simulink model "ea_model"  (Simulink 8.8)
settings: Solver=ode23  StartTime=0.0  StopTime=10  MaxStep=.01  RelTol=1e-3  AbsTol=1e-3  EnableMultiTasking=on
undefined symbols (not defined in the file): i_smn0, L_s, M, p, psi_r_al_bet0, psi_Rmn0, psi_s_al_bet0, R_r, R_s, sigma, tau_r, tau_sigma
settings Model: Creator=Niels  LastModifiedBy=Niels  ExtModeTrigMode=oneshot  ExtModeArmWhenConnect=off
settings DataIOCC: LimitDataPoints=off  SaveOutput=off  SaveTime=off
settings OptimizationCC: BlockReduction=off  BooleanDataType=off  LifeSpan=auto
settings DebuggingCC: SaveWithParameterizedLinksMsg=none  SignalResolutionControl=TryResolveAllWithWarning  MultiTaskDSMMsg=warning  MultiTaskCondExecSysMsg=none  FcnCallInpInsideContextMsg=error  StateNameClashWarn=none  StrictBusMsg=None  SFUnexpectedBacktrackingDiag=error  SFNoUnconditionalDefaultTransitionDiag=error  SFExecutionAtInitializationDiag=warning
settings HardwareCC: ProdBitPerPointer=64  ProdBitPerSizeT=64  ProdBitPerPtrDiffT=64  ProdLargestAtomicFloat=Float  ProdIntDivRoundTo=Zero  ProdEndianess=LittleEndian  ProdWordSize=64  ProdHWDeviceType=Intel->x86-64 (Windows64)  TargetUnknown=on
settings GRTTargetCC: GeneratePreprocessorConditionals=Use local settings
settings ConfigComp: CovMetricSettings=dwe  CovHtmlReporting=off  CovSaveCumulativeToWorkspaceVar=off  CovSaveSingleToWorkspaceVar=off  CovExternalEMLEnable=on

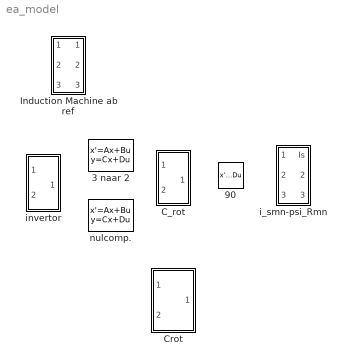
== system ea_model ==
  3 naar 2 : StateSpace  A=[]  B=[]  C=[]  D=K  X0=0  mask(Matrix gain){K=[2/3 -1/3 -1/3; 0 1/sqrt(3) -1/sqrt(3)]}
      mask prompts: K "Gain matrix:"
      mask help: Matrix Gain.
      mask Help: Multiplies input vector by entered matrix to produce output vector (y=Au).
      mask Display: disp('K')
  90 : StateSpace  A=[]  B=[]  C=[]  D=K  X0=0  mask(Matrix gain){K=[0 -1;1 0]}
      mask prompts: K "Gain matrix:"
      mask help: Matrix Gain.
      mask Help: Multiplies input vector by entered matrix to produce output vector (y=Au).
      mask Display: disp('K')
  C_rot : Subsystem
  Crot : Subsystem
  Induction Machine ab ref : Subsystem
  i_smn-psi_Rmn : Subsystem
  invertor : Subsystem
  nulcomp. : StateSpace  A=[]  B=[]  C=[]  D=K  X0=0  mask(Matrix gain){K=[1/3 1/3 1/3]}
      mask prompts: K "Gain matrix:"
      mask help: Matrix Gain.
      mask Help: Multiplies input vector by entered matrix to produce output vector (y=Au).
      mask Display: disp('K')

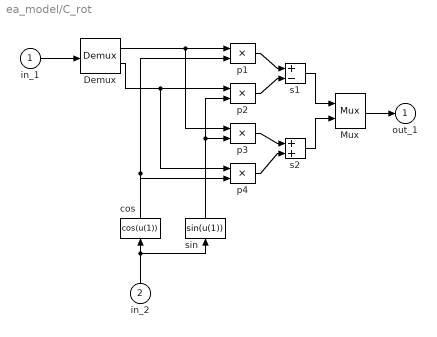
== system ea_model/C_rot ==
  in_1 : Inport
  in_2 : Inport  Port=2
  Demux : Demux  Outputs=2
  Mux : Mux  Inputs=2
  cos : Fcn  Expr=cos(u(1))
  p{1..4} (4 alike) : Product  SaturateOnIntegerOverflow=on  RndMeth=Zero  InputSameDT=on  OutDataTypeStr=Inherit: Same as first input
  s1 : Sum  Inputs=+-  SaturateOnIntegerOverflow=on  InputSameDT=on  OutDataTypeStr=Inherit: Same as first input
  s2 : Sum  SaturateOnIntegerOverflow=on  InputSameDT=on  OutDataTypeStr=Inherit: Same as first input
  sin : Fcn  Expr=sin(u(1))
  out_1 : Outport
  wires:
  s2/1 -> Mux/2
  s1/1 -> Mux/1
  p2/1 -> s1/2
  p3/1 -> s2/1
  p1/1 -> s1/1
  p4/1 -> s2/2
  in_2/1 -> cos/1, sin/1
  sin/1 -> p2/2, p3/2
  cos/1 -> p1/2, p4/2
  Demux/1 -> p1/1, p3/1
  Demux/2 -> p2/1, p4/1
  in_1/1 -> Demux/1
  Mux/1 -> out_1/1

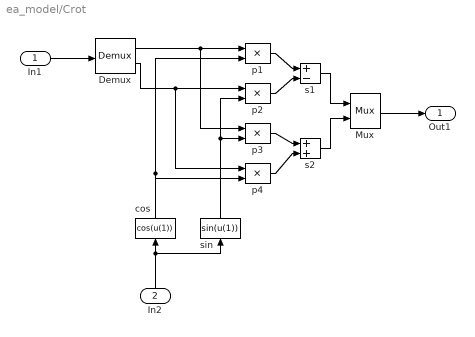
== system ea_model/Crot ==
  In1 : Inport
  In2 : Inport  Port=2
  Demux : Demux  Outputs=2
  Mux : Mux  Inputs=2
  cos : Fcn  Expr=cos(u(1))
  p{1..4} (4 alike) : Product  SaturateOnIntegerOverflow=on  RndMeth=Zero  InputSameDT=on  OutDataTypeStr=Inherit: Same as first input
  s1 : Sum  Inputs=+-  SaturateOnIntegerOverflow=on  InputSameDT=on  OutDataTypeStr=Inherit: Same as first input
  s2 : Sum  SaturateOnIntegerOverflow=on  InputSameDT=on  OutDataTypeStr=Inherit: Same as first input
  sin : Fcn  Expr=sin(u(1))
  Out1 : Outport
  wires:
  sin/1 -> p2/2, p3/2
  cos/1 -> p1/2, p4/2
  In2/1 -> cos/1, sin/1
  In1/1 -> Demux/1
  p2/1 -> s1/2
  s1/1 -> Mux/1
  Demux/1 -> p1/1, p3/1
  Mux/1 -> Out1/1
  Demux/2 -> p2/1, p4/1
  s2/1 -> Mux/2
  p3/1 -> s2/1
  p1/1 -> s1/1
  p4/1 -> s2/2

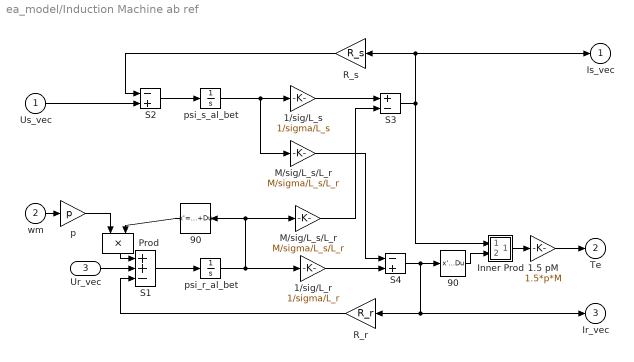
== system ea_model/Induction Machine ab ref ==
  Us_vec : Inport
  wm : Inport  Port=2
  Ur_vec : Inport  Port=3
  1.5 pM : Gain  Gain=1.5*p*M  SaturateOnIntegerOverflow=on  OutDataTypeStr=Inherit: Same as input  ParamDataTypeStr=Inherit: Same as input
  1/sig/L_r : Gain  Gain=1/sigma/L_r  SaturateOnIntegerOverflow=on  OutDataTypeStr=Inherit: Same as input  ParamDataTypeStr=Inherit: Same as input
  "1/sig/L_s " : Gain  Gain=1/sigma/L_s  SaturateOnIntegerOverflow=on  OutDataTypeStr=Inherit: Same as input  ParamDataTypeStr=Inherit: Same as input
  90 : StateSpace  A=[]  B=[]  C=[]  D=K  X0=0  mask(Matrix gain){K=[0 -1;1 0]}
      mask prompts: K "Gain matrix:"
      mask help: Matrix Gain.
      mask Help: Multiplies input vector by entered matrix to produce output vector (y=Au).
      mask Display: disp('K')
  "90 " : StateSpace  A=[]  B=[]  C=[]  D=K  X0=0  mask(Matrix gain){K=[0 -1;1 0]}
      mask prompts: K "Gain matrix:"
      mask help: Matrix Gain.
      mask Help: Multiplies input vector by entered matrix to produce output vector (y=Au).
      mask Display: disp('K')
  Inner Prod : Subsystem  mask(Dot Product){}
      mask help:
      | Inner (dot) product.
      | y=sum(u1.*u2)
      mask Help: Computes the inner (dot) product of the inputs: sum(u1.*u2).  The inputs are vectors of the same length. Output is a scalar.
      mask Display: disp('.\n')
  M/sig/L_s/L_r : Gain  Gain=M/sigma/L_s/L_r  SaturateOnIntegerOverflow=on  OutDataTypeStr=Inherit: Same as input  ParamDataTypeStr=Inherit: Same as input
  "M/sig/L_s/L_r " : Gain  Gain=M/sigma/L_s/L_r  SaturateOnIntegerOverflow=on  OutDataTypeStr=Inherit: Same as input  ParamDataTypeStr=Inherit: Same as input
  Prod : Product  SaturateOnIntegerOverflow=on  RndMeth=Zero  InputSameDT=on  OutDataTypeStr=Inherit: Same as first input
  R_r : Gain  Gain=R_r  SaturateOnIntegerOverflow=on  OutDataTypeStr=Inherit: Same as input  ParamDataTypeStr=Inherit: Same as input
  R_s : Gain  Gain=R_s  SaturateOnIntegerOverflow=on  OutDataTypeStr=Inherit: Same as input  ParamDataTypeStr=Inherit: Same as input
  S1 : Sum  Inputs=++-  SaturateOnIntegerOverflow=on  InputSameDT=on  OutDataTypeStr=Inherit: Same as first input
  S2 : Sum  Inputs=-+  SaturateOnIntegerOverflow=on  InputSameDT=on  OutDataTypeStr=Inherit: Same as first input
  S3 : Sum  Inputs=+-  SaturateOnIntegerOverflow=on  InputSameDT=on  OutDataTypeStr=Inherit: Same as first input
  S4 : Sum  Inputs=-+  SaturateOnIntegerOverflow=on  InputSameDT=on  OutDataTypeStr=Inherit: Same as first input
  p : Gain  Gain=p  SaturateOnIntegerOverflow=on  OutDataTypeStr=Inherit: Same as input  ParamDataTypeStr=Inherit: Same as input
  psi_r_al_bet : Integrator  InitialCondition=psi_r_al_bet0
  psi_s_al_bet : Integrator  InitialCondition=psi_s_al_bet0
  Is_vec : Outport
  Te : Outport  Port=2
  Ir_vec : Outport  Port=3
  wires:
  p/1 -> Prod/1
  R_r/1 -> S1/3
  Ur_vec/1 -> S1/2
  90/1 -> Prod/2
  psi_r_al_bet/1 -> 1/sig/L_r/1, "M/sig/L_s/L_r "/1, 90/1
  Prod/1 -> S1/1
  R_s/1 -> S2/1
  M/sig/L_s/L_r/1 -> S4/1
  "M/sig/L_s/L_r "/1 -> S3/2
  "1/sig/L_s "/1 -> S3/1
  1/sig/L_r/1 -> S4/2
  psi_s_al_bet/1 -> "1/sig/L_s "/1, M/sig/L_s/L_r/1
  S2/1 -> psi_s_al_bet/1
  S1/1 -> psi_r_al_bet/1
  Inner Prod/1(out_1) -> 1.5 pM/1
  "90 "/1 -> Inner Prod/2(in_2)
  S3/1 -> Is_vec/1, R_s/1, Inner Prod/1(in_1)
  Us_vec/1 -> S2/2
  wm/1 -> p/1
  1.5 pM/1 -> Te/1
  S4/1 -> Ir_vec/1, R_r/1, "90 "/1

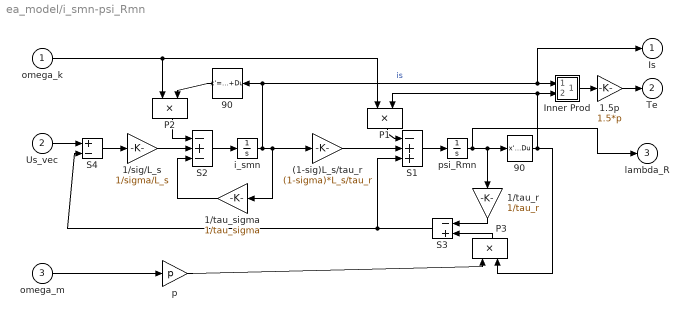
== system ea_model/i_smn-psi_Rmn ==
  omega_k : Inport
  Us_vec : Inport  Port=2
  omega_m : Inport  Port=3
  (1-sig)L_s/tau_r : Gain  Gain=(1-sigma)*L_s/tau_r  SaturateOnIntegerOverflow=on  OutDataTypeStr=Inherit: Same as input  ParamDataTypeStr=Inherit: Same as input
  1.5p : Gain  Gain=1.5*p  SaturateOnIntegerOverflow=on  OutDataTypeStr=Inherit: Same as input  ParamDataTypeStr=Inherit: Same as input
  1/sig/L_s : Gain  Gain=1/sigma/L_s  SaturateOnIntegerOverflow=on  OutDataTypeStr=Inherit: Same as input  ParamDataTypeStr=Inherit: Same as input
  1/tau_r : Gain  Gain=1/tau_r  SaturateOnIntegerOverflow=on  OutDataTypeStr=Inherit: Same as input  ParamDataTypeStr=Inherit: Same as input
  1/tau_sigma : Gain  Gain=1/tau_sigma  SaturateOnIntegerOverflow=on  OutDataTypeStr=Inherit: Same as input  ParamDataTypeStr=Inherit: Same as input
  90 : StateSpace  A=[]  B=[]  C=[]  D=K  X0=0  mask(Matrix gain){K=[0 -1;1 0]}
      mask prompts: K "Gain matrix:"
      mask help: Matrix Gain.
      mask Help: Multiplies input vector by entered matrix to produce output vector (y=Au).
      mask Display: disp('K')
  "90 " : StateSpace  A=[]  B=[]  C=[]  D=K  X0=0  mask(Matrix gain){K=[0 -1;1 0]}
      mask prompts: K "Gain matrix:"
      mask help: Matrix Gain.
      mask Help: Multiplies input vector by entered matrix to produce output vector (y=Au).
      mask Display: disp('K')
  Inner Prod : Subsystem  mask(Dot Product){}
      mask help:
      | Inner (dot) product.
      | y=sum(u1.*u2)
      mask Help: Computes the inner (dot) product of the inputs: sum(u1.*u2).  The inputs are vectors of the same length. Output is a scalar.
      mask Display: disp('.\n')
  P1 : Product  SaturateOnIntegerOverflow=on  RndMeth=Zero  InputSameDT=on  OutDataTypeStr=Inherit: Same as first input
  P2 : Product  SaturateOnIntegerOverflow=on  RndMeth=Zero  InputSameDT=on  OutDataTypeStr=Inherit: Same as first input
  P3 : Product  SaturateOnIntegerOverflow=on  RndMeth=Zero  InputSameDT=on  OutDataTypeStr=Inherit: Same as first input
  S1 : Sum  Inputs=-++  SaturateOnIntegerOverflow=on  InputSameDT=on  OutDataTypeStr=Inherit: Same as first input
  S2 : Sum  Inputs=-+-  SaturateOnIntegerOverflow=on  InputSameDT=on  OutDataTypeStr=Inherit: Same as first input
  S3 : Sum  Inputs=-+  SaturateOnIntegerOverflow=on  InputSameDT=on  OutDataTypeStr=Inherit: Same as first input
  S4 : Sum  Inputs=+-  SaturateOnIntegerOverflow=on  InputSameDT=on  OutDataTypeStr=Inherit: Same as first input
  i_smn : Integrator  InitialCondition=i_smn0
  "p " : Gain  Gain=p  SaturateOnIntegerOverflow=on  OutDataTypeStr=Inherit: Same as input  ParamDataTypeStr=Inherit: Same as input
  psi_Rmn : Integrator  InitialCondition=psi_Rmn0
  Is : Outport
  Te : Outport  Port=2
  lambda_R : Outport  Port=3
  wires:
  Inner Prod/1(out_1) -> 1.5p/1
  S3/1 -> S1/3, S4/2
  S4/1 -> 1/sig/L_s/1
  1/sig/L_s/1 -> S2/2
  90/1 -> P2/2
  P2/1 -> S2/1
  P1/1 -> S1/1
  1/tau_sigma/1 -> S2/3
  S2/1 -> i_smn/1
  (1-sig)L_s/tau_r/1 -> S1/2
  "p "/1 -> P3/1
  P3/1 -> S3/2
  1/tau_r/1 -> S3/1
  S1/1 -> psi_Rmn/1
  Us_vec/1 -> S4/1
  omega_m/1 -> "p "/1
  "90 "/1 -> P3/2, Inner Prod/2(in_2), P1/2
  omega_k/1 -> P1/1, P2/1
  i_smn/1 -> (1-sig)L_s/tau_r/1, 1/tau_sigma/1, 90/1, Inner Prod/1(in_1), Is/1  "is"
  psi_Rmn/1 -> "90 "/1, 1/tau_r/1, lambda_R/1
  1.5p/1 -> Te/1

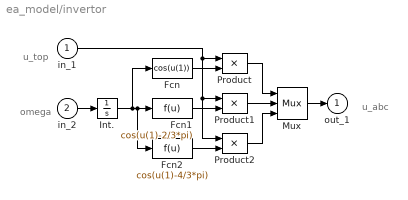
== system ea_model/invertor ==
  note: u_top
  note: omega
  note: u_abc
  in_1 : Inport
  in_2 : Inport  Port=2
  Fcn : Fcn  Expr=cos(u(1))
  Fcn1 : Fcn  Expr=cos(u(1)-2/3*pi)
  Fcn2 : Fcn  Expr=cos(u(1)-4/3*pi)
  Int. : Integrator
  Mux : Mux  Inputs=3
  Product : Product  SaturateOnIntegerOverflow=on  RndMeth=Zero  InputSameDT=on  OutDataTypeStr=Inherit: Same as first input
  Product1 : Product  SaturateOnIntegerOverflow=on  RndMeth=Zero  InputSameDT=on  OutDataTypeStr=Inherit: Same as first input
  Product2 : Product  SaturateOnIntegerOverflow=on  RndMeth=Zero  InputSameDT=on  OutDataTypeStr=Inherit: Same as first input
  out_1 : Outport
  wires:
  in_1/1 -> Product/1, Product1/1, Product2/1
  Fcn/1 -> Product/2
  Fcn1/1 -> Product1/2
  Fcn2/1 -> Product2/2
  Product1/1 -> Mux/2
  in_2/1 -> Int./1
  Int./1 -> Fcn1/1, Fcn2/1, Fcn/1
  Product/1 -> Mux/1
  Product2/1 -> Mux/3
  Mux/1 -> out_1/1

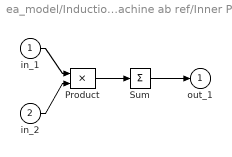
== system ea_model/Induction Machine ab ref/Inner Prod ==
  in_1 : Inport
  in_2 : Inport  Port=2
  Product : Product  SaturateOnIntegerOverflow=on  RndMeth=Zero  InputSameDT=on  OutDataTypeStr=Inherit: Same as first input
  Sum : Sum  Inputs=+  SaturateOnIntegerOverflow=on  InputSameDT=on  OutDataTypeStr=Inherit: Same as first input
  out_1 : Outport
  wires:
  in_2/1 -> Product/2
  in_1/1 -> Product/1
  Product/1 -> Sum/1
  Sum/1 -> out_1/1

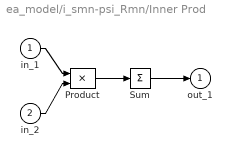
== system ea_model/i_smn-psi_Rmn/Inner Prod ==
  in_1 : Inport
  in_2 : Inport  Port=2
  Product : Product  SaturateOnIntegerOverflow=on  RndMeth=Zero  InputSameDT=on  OutDataTypeStr=Inherit: Same as first input
  Sum : Sum  Inputs=+  SaturateOnIntegerOverflow=on  InputSameDT=on  OutDataTypeStr=Inherit: Same as first input
  out_1 : Outport
  wires:
  in_2/1 -> Product/2
  in_1/1 -> Product/1
  Product/1 -> Sum/1
  Sum/1 -> out_1/1
